simulink model "scheme"  (R2024a)
settings: Solver=VariableStepAuto  StartTime=0.0  StopTime=100  RelTol=1e-3
InitFcn:
  | a0=-11; a1=-1; b0=3;
  | A=[0 1; -a0 -a1];
  | b=[0; b0];
  | am0=10.24; am1=6.4;
  | Am=[0 1; -am0 -am1];
  | bm=[0; am0];
  | theta1=(a0-am0)/b0;
  | theta2=(a1-am1)/b0;
  | theta=[theta1; theta2];
  | kappa=b0/am0;
  | Q=eye(2);
  | P=lyap(Am',Q);
settings Model: Creator=User  LastModifiedBy=User

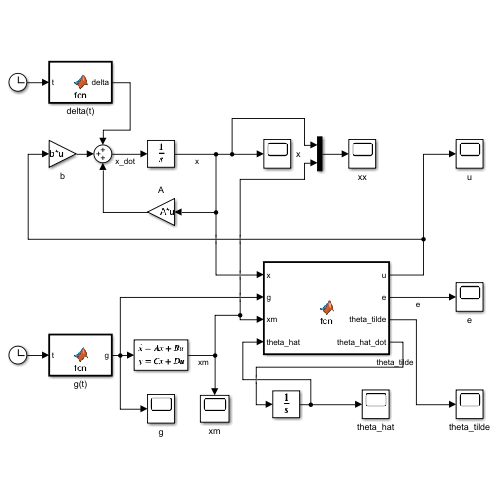
[thumbnail: Simulink's stored preview of the top-level diagram]
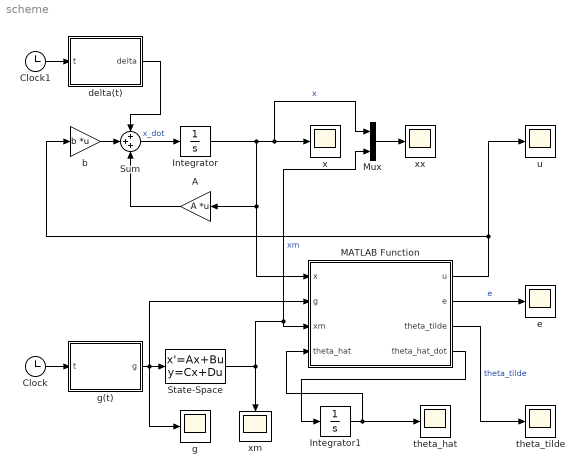
== system scheme ==
  A : Gain  Gain=A  Multiplication=Matrix(K*u)
  Clock : Clock
  Clock1 : Clock
  Integrator : Integrator  InitialCondition=[0; 0]
  Integrator1 : Integrator  InitialCondition=[0; 0]
  MATLAB Function : MATLAB Function  TreatAsAtomicUnit=on
  Mux : Mux  Inputs=2
  State-Space : StateSpace  A=Am  B=bm  C=eye(2)  D=[0;0]  InitialCondition=[0;0]
  Sum : Sum  Inputs=+++
  b : Gain  Gain=b  Multiplication=Matrix(K*u)
  delta(t) : MATLAB Function  TreatAsAtomicUnit=on
  e : Scope
  g : Scope
  g(t) : MATLAB Function  TreatAsAtomicUnit=on
  theta_hat : Scope
  theta_tilde : Scope
  u : Scope
  x : Scope
  xm : Scope
  xx : Scope
  wires:
  Integrator/1 -> Mux/1, x/1, MATLAB Function/1(x), A/1  "x"
  Sum/1 -> Integrator/1  "x_dot"
  g(t)/1(g) -> State-Space/1, g/1, MATLAB Function/2(g)
  Clock/1 -> g(t)/1(t)
  State-Space/1 -> Mux/2, MATLAB Function/3(xm), xm/1  "xm"
  MATLAB Function/4(theta_hat_dot) -> Integrator1/1
  Integrator1/1 -> MATLAB Function/4(theta_hat), theta_hat/1
  MATLAB Function/3(theta_tilde) -> theta_tilde/1  "theta_tilde"
  MATLAB Function/2(e) -> e/1  "e"
  MATLAB Function/1(u) -> u/1, b/1
  Mux/1 -> xx/1
  b/1 -> Sum/2
  A/1 -> Sum/3
  Clock1/1 -> delta(t)/1(t)
  delta(t)/1(delta) -> Sum/1

== matlab function scheme/MATLAB Function ==
  data: x input; g input; xm input; theta_hat input; u output; e output; kappa parameter; b parameter; theta parameter; P parameter; theta_tilde output; theta_hat_dot output
function [u, e, theta_tilde, theta_hat_dot] = fcn(x, g, xm, theta_hat, kappa, b, theta, P)
gamma=100; %10, 100
sigma=0.1; %1, 0.1

e=xm-x;
u=theta_hat'*x+1/kappa*g;
theta_tilde = theta - theta_hat;
theta_hat_dot = -sigma*theta_hat+gamma*x*b'*P*e;

== matlab function scheme/g(t) ==
  data: t input; g output
function g = fcn(t)

g = sign(sin(0.5*t))+3; %sign(sin(0.5*t))+3

== matlab function scheme/delta(t) ==
  data: t input; delta output
function delta = fcn(t)
% [0.6*sin(10*t)+0.1*sin(50*t); 0.5*cos(12*t)+0.2*sin(30*t)]
delta = [0.6*sin(10*t)+0.1*sin(50*t); 0.5*cos(12*t)+0.2*sin(30*t)];
